simulink model "kalman_filter"  (R2015b)
settings: Solver=VariableStepAuto  StartTime=0.0  StopTime=10.0  RelTol=1e-3
values from neighbouring files (symbols this model uses):
  Ad = sysd.a    [dp_EKF_script.m]    (also in dp_kalman_script.m; dp_real_vs_lin_script.m; dp_statefeedback_script.m)
  Bd = sysd.b    [dp_EKF_script.m]    (also in dp_kalman_script.m; dp_real_vs_lin_script.m; dp_statefeedback_script.m)
  Cd_kalman = Cd(1,:)    [dp_kalman_script.m]    (also in dp_real_vs_lin_script.m)
  x0 = [phi1_0; dphi1_0; phi2_0; dphi2_0]    [dp_EKF_script.m]    (also in dp_UKF_script.m; dp_kalman_script.m; dp_real_vs_lin_script.m; dp_statefeedback_script.m)
settings Model: Creator=serov  LastModifiedBy=serov

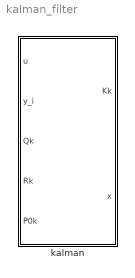
== system kalman_filter ==
  kalman : MATLAB Function  TreatAsAtomicUnit=on

== matlab function kalman_filter/kalman ==
  data: u input; y_i input; Qk input size=[4 4]; Rk input; Ad parameter; Bd parameter; Cd_kalman parameter; Kk output size=[4 1]; x output size=[4 1]; x0 parameter; P0k input
function [Kk, x] = fcn(u, y_i, Qk, Rk, Ad, Bd, Cd_kalman, x0, P0k)
%#codegen
persistent x_p P_p
%% Initialisierung im ersten Zeitschritt wird nur einmal aufgerufen
if isempty(x_p)
    x_p = zeros(4,1);
    x = zeros(4,1);
% korrekte Initialisierung
%    x_p = x0;    
%    x = x_p;
    P_p = P0k;
    Kk = zeros(4,1); 
else
%% Discrete Time update: prediction
x = Ad*x_p + Bd * u;
P = Ad*P_p*Ad' + Qk;
%% Measurement update: correction
Kk = P*Cd_kalman' *(Cd_kalman*P*Cd_kalman' + Rk)^(-1);
x = x + Kk * (y_i - Cd_kalman*x);
P = (eye(4) - Kk *Cd_kalman)*P;
x_p = x;
P_p = P;
end
